simulink model "COSTEP_Auto"  (R2024b)
settings: Solver=FixedStepAuto  StartTime=0.0  StopTime=25  FixedStep=1/3600  RelTol=1e-3
model workspace (MAT data in the model file):
  AD : Simulink.Parameter (value not decoded)
  AG : Simulink.Parameter (value not decoded)
  AH : Simulink.Parameter (value not decoded)
  AV : Simulink.Parameter (value not decoded)
  AVP : Simulink.Parameter (value not decoded)
  BCHL : Simulink.Parameter (value not decoded)
  BCHV : Simulink.Parameter (value not decoded)
  BD : Simulink.Parameter (value not decoded)
  BG : Simulink.Parameter (value not decoded)
  BH : Simulink.Parameter (value not decoded)
  BVP : Simulink.Parameter (value not decoded)
  CD : Simulink.Parameter (value not decoded)
  CG : Simulink.Parameter (value not decoded)
  CH : Simulink.Parameter (value not decoded)
  CVP : Simulink.Parameter (value not decoded)
  ISV : Simulink.Parameter (value not decoded)
  XMW : Simulink.Parameter (value not decoded)
  XNS : Simulink.Parameter (value not decoded)
  XNS2 : Simulink.Parameter (value not decoded)
  XNS3 : Simulink.Parameter (value not decoded)
  XNSE : Simulink.Parameter (value not decoded)
values from neighbouring files (symbols this model uses):
  DD = SimData{4,1}{1,2}    [Auto_run_COSTEP.m]    (also in Run_COSTEP.m)
  G = SimData{2,1}(j,2)    [Auto_run_COSTEP.m]    (also in G.mat = [4243534565 7854912354 3456432354 1731738903 4346024432 5784; Run_COSTEP.m)
  IDV = SimData{3,1}(1:20,j)    [Auto_run_COSTEP.m]    (also in IDV.mat = [0 0 0 0 0 0 0 0 0 0 0 0 ... (812 elements, 28x29)]; Run_COSTEP.m = SimData{3,1}(1:28,j))
symbols that are objects in the model workspace (value not decoded): AD, AG, AH, AV, AVP, BD, BG, BH, BVP, CD, CG, CH, CVP, XMW, XNS, XNS2, XNS3, XNSE
undefined symbols (not defined in the file or in its folder): magnitude, msgbox, SETPT, XMEAS, XMV
libraries: mylib x304, dspindex x31
(part 8 of 13)

== system COSTEP_Auto/Mixing Zone/Stream 6/Subsystem/If Action Subsystem1 ==
  In1 : Inport
  Action Port : ActionPort  ActionPortLabel=else
  Out1 : Outport  VectorParamsAs1DForOutWhenUnconnected=off
  wires:
  In1/1 -> Out1/1

== system COSTEP_Auto/Process Measurements/Feed Streams/D Feed/XMWS(1) Molecular weight of Stream 1 lb//lb-mol ==
  XST(I,1) : Inport
  Product : Product
  Sum of Elements : Sum  Inputs=+
  "XMW(I) Molecular weight of components lb/lb-mol " : Constant  Value=XMW
  XMWS(1) : Outport  VectorParamsAs1DForOutWhenUnconnected=off
  wires:
  Sum of Elements/1 -> XMWS(1)/1
  Product/1 -> Sum of Elements/1
  XST(I,1)/1 -> Product/1
  "XMW(I) Molecular weight of components lb/lb-mol "/1 -> Product/2

== system COSTEP_Auto/Process Measurements/Feed Streams/E Feed/XMWS(2) Molecular weight of Stream 2 lb//lb-mol ==
  XST(I,2) : Inport
  Product : Product
  Sum of Elements : Sum  Inputs=+
  "XMW(I) Molecular weight of components lb/lb-mol " : Constant  Value=XMW
  XMWS(2) : Outport  VectorParamsAs1DForOutWhenUnconnected=off
  wires:
  Sum of Elements/1 -> XMWS(2)/1
  Product/1 -> Sum of Elements/1
  XST(I,2)/1 -> Product/1
  "XMW(I) Molecular weight of components lb/lb-mol "/1 -> Product/2

== system COSTEP_Auto/Process Measurements/Product analysis/Subsystem/Subsystem ==
  XST : Inport
  Constant : Constant  Value=100
  Multiport Selector : dspindex/Multiport Selector  rowsOrCols=Rows  idxCellArray={4,5,6,7,8}  idxErrMode=Clip Index
  XCMP(37) : Product
  XCMP(38) : Product
  XCMP(39) : Product
  XCMP(40) : Product
  XCMP(41) : Product
  "XCMP(37) " : Outport  VectorParamsAs1DForOutWhenUnconnected=off
  "XCMP(38) " : Outport  Port=2  VectorParamsAs1DForOutWhenUnconnected=off
  "XCMP(39) " : Outport  Port=3  VectorParamsAs1DForOutWhenUnconnected=off
  "XCMP(40) " : Outport  Port=4  VectorParamsAs1DForOutWhenUnconnected=off
  "XCMP(41) " : Outport  Port=5  VectorParamsAs1DForOutWhenUnconnected=off
  wires:
  Constant/1 -> XCMP(38)/2, XCMP(40)/2, XCMP(41)/2, XCMP(39)/2, XCMP(37)/2
  Multiport Selector/1 -> XCMP(37)/1
  XCMP(37)/1 -> "XCMP(37) "/1  "XCMP(37)"
  Multiport Selector/5 -> XCMP(41)/1
  XCMP(39)/1 -> "XCMP(39) "/1  "XCMP(39)"
  XST/1 -> Multiport Selector/1
  Multiport Selector/4 -> XCMP(40)/1
  Multiport Selector/2 -> XCMP(38)/1
  Multiport Selector/3 -> XCMP(39)/1
  XCMP(38)/1 -> "XCMP(38) "/1  "XCMP(38)"
  XCMP(41)/1 -> "XCMP(41) "/1  "XCMP(41)"
  XCMP(40)/1 -> "XCMP(40) "/1  "XCMP(40)"

== system COSTEP_Auto/Process Measurements/Purge gas analysis/Subsystem/Subsystem ==
  XST : Inport
  Constant : Constant  Value=100
  Multiport Selector : dspindex/Multiport Selector  rowsOrCols=Rows  idxCellArray={ 1,2,3,4,5,6,7,8}  idxErrMode=Clip Index
  XCMP(29) : Product
  XCMP(30) : Product
  XCMP(31) : Product
  XCMP(32) : Product
  XCMP(33) : Product
  XCMP(34) : Product
  XCMP(35) : Product
  XCMP(36) : Product
  "XCMP(29) " : Outport  VectorParamsAs1DForOutWhenUnconnected=off
  "XCMP(30) " : Outport  Port=2  VectorParamsAs1DForOutWhenUnconnected=off
  "XCMP(31) " : Outport  Port=3  VectorParamsAs1DForOutWhenUnconnected=off
  "XCMP(32) " : Outport  Port=4  VectorParamsAs1DForOutWhenUnconnected=off
  "XCMP(33) " : Outport  Port=5  VectorParamsAs1DForOutWhenUnconnected=off
  "XCMP(34) " : Outport  Port=6  VectorParamsAs1DForOutWhenUnconnected=off
  "XCMP(35) " : Outport  Port=7  VectorParamsAs1DForOutWhenUnconnected=off
  "XCMP(36) " : Outport  Port=8  VectorParamsAs1DForOutWhenUnconnected=off
  wires:
  XCMP(32)/1 -> "XCMP(32) "/1  "XCMP(32)"
  Multiport Selector/6 -> XCMP(34)/1
  Multiport Selector/8 -> XCMP(36)/1
  XCMP(29)/1 -> "XCMP(29) "/1  "XCMP(29)"
  Multiport Selector/5 -> XCMP(33)/1
  Multiport Selector/7 -> XCMP(35)/1
  XCMP(30)/1 -> "XCMP(30) "/1  "XCMP(30)"
  Multiport Selector/1 -> XCMP(29)/1
  Multiport Selector/3 -> XCMP(31)/1
  Constant/1 -> XCMP(32)/2, XCMP(36)/2, XCMP(35)/2, XCMP(34)/2, XCMP(33)/2, XCMP(31)/2, XCMP(30)/2, XCMP(29)/2
  XCMP(33)/1 -> "XCMP(33) "/1  "XCMP(33)"
  Multiport Selector/4 -> XCMP(32)/1
  XST/1 -> Multiport Selector/1
  Multiport Selector/2 -> XCMP(30)/1
  XCMP(31)/1 -> "XCMP(31) "/1  "XCMP(31)"
  XCMP(35)/1 -> "XCMP(35) "/1  "XCMP(35)"
  XCMP(36)/1 -> "XCMP(36) "/1  "XCMP(36)"
  XCMP(34)/1 -> "XCMP(34) "/1  "XCMP(34)"

== system COSTEP_Auto/Process Measurements/Reactor feed analysis/Subsystem/Subsystem ==
  XST : Inport
  Constant : Constant  Value=100
  Multiport Selector : dspindex/Multiport Selector  rowsOrCols=Rows  idxCellArray={ 1,2,3,4,5,6,}  idxErrMode=Clip Index
  XCMP(23) : Product
  XCMP(24) : Product
  XCMP(25) : Product
  XCMP(26) : Product
  XCMP(27) : Product
  XCMP(28) : Product
  XCMP(23)1 : Outport  VectorParamsAs1DForOutWhenUnconnected=off
  XCMP(24)1 : Outport  Port=2  VectorParamsAs1DForOutWhenUnconnected=off
  XCMP(25)1 : Outport  Port=3  VectorParamsAs1DForOutWhenUnconnected=off
  XCMP(26)1 : Outport  Port=4  VectorParamsAs1DForOutWhenUnconnected=off
  XCMP(27)1 : Outport  Port=5  VectorParamsAs1DForOutWhenUnconnected=off
  XCMP(28)1 : Outport  Port=6  VectorParamsAs1DForOutWhenUnconnected=off
  wires:
  Multiport Selector/1 -> XCMP(23)/1  "XST(1;7)"
  Multiport Selector/4 -> XCMP(26)/1  "XST(4;7)"
  Constant/1 -> XCMP(26)/2, XCMP(28)/2, XCMP(27)/2, XCMP(25)/2, XCMP(24)/2, XCMP(23)/2
  Multiport Selector/2 -> XCMP(24)/1  "XST(2;7)"
  XST/1 -> Multiport Selector/1
  Multiport Selector/6 -> XCMP(28)/1  "XST(6:7)"
  Multiport Selector/3 -> XCMP(25)/1  "XST(3;7)"
  XCMP(23)/1 -> XCMP(23)1/1  "XCMP(23)"
  Multiport Selector/5 -> XCMP(27)/1  "XST(5;7)"
  XCMP(25)/1 -> XCMP(25)1/1  "XCMP(25)"
  XCMP(26)/1 -> XCMP(26)1/1  "XCMP(26)"
  XCMP(24)/1 -> XCMP(24)1/1  "XCMP(24)"
  XCMP(27)/1 -> XCMP(27)1/1  "XCMP(27)"
  XCMP(28)/1 -> XCMP(28)1/1  "XCMP(28)"

== system COSTEP_Auto/Random number generator/Disturbances I=1-9/Subsystem1/DIST(2)_0 ==
  BDIST(2) : Constant  Value=0
  Bus Creator : BusCreator  Inputs=6
  CDIST(2) : Constant  Value=0
  DDIST(2) : Constant  Value=0
  SZERO(2) : Constant  Value=0.005
  TENXT(2) : Constant  Value=0.1
  TLAST(2) : Constant  Value=0
  DIST : Outport  VectorParamsAs1DForOutWhenUnconnected=off
  wires:
  Bus Creator/1 -> DIST/1
  TENXT(2)/1 -> Bus Creator/5  "TNEXT"
  SZERO(2)/1 -> Bus Creator/1  "ADIST"
  TLAST(2)/1 -> Bus Creator/6  "TLAST"
  DDIST(2)/1 -> Bus Creator/4  "DDIST"
  BDIST(2)/1 -> Bus Creator/2  "BDIST"
  CDIST(2)/1 -> Bus Creator/3  "CDIST"

== system COSTEP_Auto/Random number generator/Disturbances I=1-9/Subsystem1/Subsystem ==
  Bus Creator : BusCreator  Inputs=5
  HSPAN(2) : Constant  Value=0.7
  HZERO(2) : Constant
  SPSPAN(2) : Constant  Value=0
  SSPAN(2) : Constant  Value=0.003
  SZERO(2) : Constant  Value=0.005
  Out1 : Outport  VectorParamsAs1DForOutWhenUnconnected=off
  wires:
  SSPAN(2)/1 -> Bus Creator/3  "SSPAN"
  HSPAN(2)/1 -> Bus Creator/1  "HSPAN"
  Bus Creator/1 -> Out1/1
  SPSPAN(2)/1 -> Bus Creator/5  "SPSPAN"
  HZERO(2)/1 -> Bus Creator/2  "HZERO"
  SZERO(2)/1 -> Bus Creator/4  "SZERO"

== system COSTEP_Auto/Random number generator/Disturbances I=1-9/Subsystem10/DIST(1)_0 ==
  BDIST(1) : Constant  Value=0
  Bus Creator : BusCreator  Inputs=6
  CDIST(1) : Constant  Value=0
  DDIST(1) : Constant  Value=0
  SZERO(1) : Constant  Value=0.485
  TENXT(1) : Constant  Value=0.1
  TLAST(1) : Constant  Value=0
  DIST : Outport  VectorParamsAs1DForOutWhenUnconnected=off
  wires:
  Bus Creator/1 -> DIST/1
  TENXT(1)/1 -> Bus Creator/5  "TNEXT"
  SZERO(1)/1 -> Bus Creator/1  "ADIST"
  TLAST(1)/1 -> Bus Creator/6  "TLAST"
  DDIST(1)/1 -> Bus Creator/4  "DDIST"
  BDIST(1)/1 -> Bus Creator/2  "BDIST"
  CDIST(1)/1 -> Bus Creator/3  "CDIST"

== system COSTEP_Auto/Random number generator/Disturbances I=1-9/Subsystem10/Subsystem ==
  Bus Creator : BusCreator  Inputs=5
  HSPAN(1) : Constant  Value=0.2
  HZERO(1) : Constant  Value=0.5
  SPSPAN(1) : Constant  Value=0
  SSPAN(1) : Constant  Value=0.03
  SZERO(1) : Constant  Value=0.485
  Out1 : Outport  VectorParamsAs1DForOutWhenUnconnected=off
  wires:
  SSPAN(1)/1 -> Bus Creator/3  "SSPAN"
  HSPAN(1)/1 -> Bus Creator/1  "HSPAN"
  Bus Creator/1 -> Out1/1
  SPSPAN(1)/1 -> Bus Creator/5  "SPSPAN"
  HZERO(1)/1 -> Bus Creator/2  "HZERO"
  SZERO(1)/1 -> Bus Creator/4  "SZERO"

== system COSTEP_Auto/Random number generator/Disturbances I=1-9/Subsystem2/DIST(3)_0 ==
  BDIST(3) : Constant  Value=0
  Bus Creator : BusCreator  Inputs=6
  CDIST(3) : Constant  Value=0
  DDIST(3) : Constant  Value=0
  SZERO(3) : Constant  Value=45
  TENXT(3) : Constant  Value=0.1
  TLAST(3) : Constant  Value=0
  DIST : Outport  VectorParamsAs1DForOutWhenUnconnected=off
  wires:
  Bus Creator/1 -> DIST/1
  TENXT(3)/1 -> Bus Creator/5  "TNEXT"
  SZERO(3)/1 -> Bus Creator/1  "ADIST"
  TLAST(3)/1 -> Bus Creator/6  "TLAST"
  DDIST(3)/1 -> Bus Creator/4  "DDIST"
  BDIST(3)/1 -> Bus Creator/2  "BDIST"
  CDIST(3)/1 -> Bus Creator/3  "CDIST"

== system COSTEP_Auto/Random number generator/Disturbances I=1-9/Subsystem2/Subsystem ==
  Bus Creator : BusCreator  Inputs=5
  HSPAN(3) : Constant  Value=0.25
  HZERO(3) : Constant  Value=0.5
  SPSPAN(3) : Constant  Value=0
  SSPAN(3) : Constant  Value=10
  SZERO(3) : Constant  Value=45
  Out1 : Outport  VectorParamsAs1DForOutWhenUnconnected=off
  wires:
  SSPAN(3)/1 -> Bus Creator/3  "SSPAN"
  HSPAN(3)/1 -> Bus Creator/1  "HSPAN"
  Bus Creator/1 -> Out1/1
  SPSPAN(3)/1 -> Bus Creator/5  "SPSPAN"
  HZERO(3)/1 -> Bus Creator/2  "HZERO"
  SZERO(3)/1 -> Bus Creator/4  "SZERO"

== system COSTEP_Auto/Random number generator/Disturbances I=1-9/Subsystem3/DIST(4)_0 ==
  BDIST(4) : Constant  Value=0
  Bus Creator : BusCreator  Inputs=6
  CDIST(4) : Constant  Value=0
  DDIST(4) : Constant  Value=0
  SZERO(4) : Constant  Value=45
  TENXT(4) : Constant  Value=0.1
  TLAST(4) : Constant  Value=0
  DIST : Outport  VectorParamsAs1DForOutWhenUnconnected=off
  wires:
  Bus Creator/1 -> DIST/1
  TENXT(4)/1 -> Bus Creator/5  "TNEXT"
  SZERO(4)/1 -> Bus Creator/1  "ADIST"
  TLAST(4)/1 -> Bus Creator/6  "TLAST"
  DDIST(4)/1 -> Bus Creator/4  "DDIST"
  BDIST(4)/1 -> Bus Creator/2  "BDIST"
  CDIST(4)/1 -> Bus Creator/3  "CDIST"

== system COSTEP_Auto/Random number generator/Disturbances I=1-9/Subsystem3/Subsystem ==
  Bus Creator : BusCreator  Inputs=5
  HSPAN(4) : Constant  Value=0.7
  HZERO(4) : Constant
  SPSPAN(4) : Constant  Value=0
  SSPAN(4) : Constant  Value=10
  SZERO(4) : Constant  Value=45
  Out1 : Outport  VectorParamsAs1DForOutWhenUnconnected=off
  wires:
  SSPAN(4)/1 -> Bus Creator/3  "SSPAN"
  HSPAN(4)/1 -> Bus Creator/1  "HSPAN"
  Bus Creator/1 -> Out1/1
  SPSPAN(4)/1 -> Bus Creator/5  "SPSPAN"
  HZERO(4)/1 -> Bus Creator/2  "HZERO"
  SZERO(4)/1 -> Bus Creator/4  "SZERO"

== system COSTEP_Auto/Random number generator/Disturbances I=1-9/Subsystem4/DIST(5)_0 ==
  BDIST(5) : Constant  Value=0
  Bus Creator : BusCreator  Inputs=6
  CDIST(5) : Constant  Value=0
  DDIST(5) : Constant  Value=0
  SZERO(5) : Constant  Value=35
  TENXT(5) : Constant  Value=0.1
  TLAST(5) : Constant  Value=0
  DIST : Outport  VectorParamsAs1DForOutWhenUnconnected=off
  wires:
  Bus Creator/1 -> DIST/1
  TENXT(5)/1 -> Bus Creator/5  "TNEXT"
  SZERO(5)/1 -> Bus Creator/1  "ADIST"
  TLAST(5)/1 -> Bus Creator/6  "TLAST"
  DDIST(5)/1 -> Bus Creator/4  "DDIST"
  BDIST(5)/1 -> Bus Creator/2  "BDIST"
  CDIST(5)/1 -> Bus Creator/3  "CDIST"

== system COSTEP_Auto/Random number generator/Disturbances I=1-9/Subsystem4/Subsystem ==
  Bus Creator : BusCreator  Inputs=5
  HSPAN(5) : Constant  Value=0.15
  HZERO(5) : Constant  Value=0.25
  SPSPAN(5) : Constant  Value=0
  SSPAN(5) : Constant  Value=10
  SZERO(5) : Constant  Value=35
  Out1 : Outport  VectorParamsAs1DForOutWhenUnconnected=off
  wires:
  SSPAN(5)/1 -> Bus Creator/3  "SSPAN"
  HSPAN(5)/1 -> Bus Creator/1  "HSPAN"
  Bus Creator/1 -> Out1/1
  SPSPAN(5)/1 -> Bus Creator/5  "SPSPAN"
  HZERO(5)/1 -> Bus Creator/2  "HZERO"
  SZERO(5)/1 -> Bus Creator/4  "SZERO"

== system COSTEP_Auto/Random number generator/Disturbances I=1-9/Subsystem5/DIST(6)_0 ==
  BDIST(6) : Constant  Value=0
  Bus Creator : BusCreator  Inputs=6
  CDIST(6) : Constant  Value=0
  DDIST(6) : Constant  Value=0
  SZERO(6) : Constant  Value=40
  TENXT(6) : Constant  Value=0.1
  TLAST(6) : Constant  Value=0
  DIST : Outport  VectorParamsAs1DForOutWhenUnconnected=off
  wires:
  Bus Creator/1 -> DIST/1
  TENXT(6)/1 -> Bus Creator/5  "TNEXT"
  SZERO(6)/1 -> Bus Creator/1  "ADIST"
  TLAST(6)/1 -> Bus Creator/6  "TLAST"
  DDIST(6)/1 -> Bus Creator/4  "DDIST"
  BDIST(6)/1 -> Bus Creator/2  "BDIST"
  CDIST(6)/1 -> Bus Creator/3  "CDIST"

== system COSTEP_Auto/Random number generator/Disturbances I=1-9/Subsystem5/Subsystem ==
  Bus Creator : BusCreator  Inputs=5
  HSPAN(6) : Constant  Value=0.15
  HZERO(6) : Constant  Value=0.25
  SPSPAN(6) : Constant  Value=0
  SSPAN(6) : Constant  Value=10
  SZERO(6) : Constant  Value=40
  Out1 : Outport  VectorParamsAs1DForOutWhenUnconnected=off
  wires:
  SSPAN(6)/1 -> Bus Creator/3  "SSPAN"
  HSPAN(6)/1 -> Bus Creator/1  "HSPAN"
  Bus Creator/1 -> Out1/1
  SPSPAN(6)/1 -> Bus Creator/5  "SPSPAN"
  HZERO(6)/1 -> Bus Creator/2  "HZERO"
  SZERO(6)/1 -> Bus Creator/4  "SZERO"

== system COSTEP_Auto/Random number generator/Disturbances I=1-9/Subsystem6/DIST(7)_0 ==
  BDIST(7) : Constant  Value=0
  Bus Creator : BusCreator  Inputs=6
  CDIST(7) : Constant  Value=0
  DDIST(7) : Constant  Value=0
  SZERO(7) : Constant
  TENXT(7) : Constant  Value=0.1
  TLAST(7) : Constant  Value=0
  DIST : Outport  VectorParamsAs1DForOutWhenUnconnected=off
  wires:
  Bus Creator/1 -> DIST/1
  TENXT(7)/1 -> Bus Creator/5  "TNEXT"
  SZERO(7)/1 -> Bus Creator/1  "ADIST"
  TLAST(7)/1 -> Bus Creator/6  "TLAST"
  DDIST(7)/1 -> Bus Creator/4  "DDIST"
  BDIST(7)/1 -> Bus Creator/2  "BDIST"
  CDIST(7)/1 -> Bus Creator/3  "CDIST"

== system COSTEP_Auto/Random number generator/Disturbances I=1-9/Subsystem6/Subsystem ==
  Bus Creator : BusCreator  Inputs=5
  HSPAN(7) : Constant
  HZERO(7) : Constant  Value=2
  SPSPAN(7) : Constant  Value=0
  SSPAN(7) : Constant  Value=0.25
  SZERO(7) : Constant
  Out1 : Outport  VectorParamsAs1DForOutWhenUnconnected=off
  wires:
  SSPAN(7)/1 -> Bus Creator/3  "SSPAN"
  HSPAN(7)/1 -> Bus Creator/1  "HSPAN"
  Bus Creator/1 -> Out1/1
  SPSPAN(7)/1 -> Bus Creator/5  "SPSPAN"
  HZERO(7)/1 -> Bus Creator/2  "HZERO"
  SZERO(7)/1 -> Bus Creator/4  "SZERO"

== system COSTEP_Auto/Random number generator/Disturbances I=1-9/Subsystem7/DIST(8)_0 ==
  BDIST(8) : Constant  Value=0
  Bus Creator : BusCreator  Inputs=6
  CDIST(8) : Constant  Value=0
  DDIST(8) : Constant  Value=0
  SZERO(8) : Constant
  TENXT(8) : Constant  Value=0.1
  TLAST(8) : Constant  Value=0
  DIST : Outport  VectorParamsAs1DForOutWhenUnconnected=off
  wires:
  Bus Creator/1 -> DIST/1
  TENXT(8)/1 -> Bus Creator/5  "TNEXT"
  SZERO(8)/1 -> Bus Creator/1  "ADIST"
  TLAST(8)/1 -> Bus Creator/6  "TLAST"
  DDIST(8)/1 -> Bus Creator/4  "DDIST"
  BDIST(8)/1 -> Bus Creator/2  "BDIST"
  CDIST(8)/1 -> Bus Creator/3  "CDIST"

== system COSTEP_Auto/Random number generator/Disturbances I=1-9/Subsystem7/Subsystem ==
  Bus Creator : BusCreator  Inputs=5
  HSPAN(8) : Constant
  HZERO(8) : Constant  Value=2
  SPSPAN(8) : Constant  Value=0
  SSPAN(8) : Constant  Value=0.25
  SZERO(8) : Constant
  Out1 : Outport  VectorParamsAs1DForOutWhenUnconnected=off
  wires:
  SSPAN(8)/1 -> Bus Creator/3  "SSPAN"
  HSPAN(8)/1 -> Bus Creator/1  "HSPAN"
  Bus Creator/1 -> Out1/1
  SPSPAN(8)/1 -> Bus Creator/5  "SPSPAN"
  HZERO(8)/1 -> Bus Creator/2  "HZERO"
  SZERO(8)/1 -> Bus Creator/4  "SZERO"

== system COSTEP_Auto/Random number generator/Disturbances I=1-9/Subsystem8/DIST(9)_0 ==
  BDIST(9) : Constant  Value=0
  Bus Creator : BusCreator  Inputs=6
  CDIST(9) : Constant  Value=0
  DDIST(9) : Constant  Value=0
  SZERO(9) : Constant  Value=0
  TENXT(9) : Constant  Value=0.1
  TLAST(9) : Constant  Value=0
  DIST : Outport  VectorParamsAs1DForOutWhenUnconnected=off
  wires:
  Bus Creator/1 -> DIST/1
  TENXT(9)/1 -> Bus Creator/5  "TNEXT"
  SZERO(9)/1 -> Bus Creator/1  "ADIST"
  TLAST(9)/1 -> Bus Creator/6  "TLAST"
  DDIST(9)/1 -> Bus Creator/4  "DDIST"
  BDIST(9)/1 -> Bus Creator/2  "BDIST"
  CDIST(9)/1 -> Bus Creator/3  "CDIST"

== system COSTEP_Auto/Random number generator/Disturbances I=1-9/Subsystem8/Subsystem ==
  Bus Creator : BusCreator  Inputs=5
  HSPAN(9) : Constant  Value=0.4
  HZERO(9) : Constant  Value=0.5
  SPSPAN(9) : Constant  Value=0
  SSPAN(9) : Constant  Value=0.25
  SZERO(9) : Constant  Value=0
  Out1 : Outport  VectorParamsAs1DForOutWhenUnconnected=off
  wires:
  SSPAN(9)/1 -> Bus Creator/3  "SSPAN"
  HSPAN(9)/1 -> Bus Creator/1  "HSPAN"
  Bus Creator/1 -> Out1/1
  SPSPAN(9)/1 -> Bus Creator/5  "SPSPAN"
  HZERO(9)/1 -> Bus Creator/2  "HZERO"
  SZERO(9)/1 -> Bus Creator/4  "SZERO"

== system COSTEP_Auto/Random number generator/Disturbances I=10-12/Subsystem1/DIST(11)_0 ==
  BDIST(11) : Constant  Value=0
  Bus Creator : BusCreator  Inputs=6
  CDIST(11) : Constant  Value=0
  DDIST(11) : Constant  Value=0
  SZERO(11) : Constant  Value=0
  TENXT(11) : Constant  Value=0.1
  TLAST(11) : Constant  Value=0
  DIST_0 : Outport  VectorParamsAs1DForOutWhenUnconnected=off
  wires:
  Bus Creator/1 -> DIST_0/1
  TENXT(11)/1 -> Bus Creator/5  "TNEXT"
  SZERO(11)/1 -> Bus Creator/1  "ADIST"
  TLAST(11)/1 -> Bus Creator/6  "TLAST"
  DDIST(11)/1 -> Bus Creator/4  "DDIST"
  BDIST(11)/1 -> Bus Creator/2  "BDIST"
  CDIST(11)/1 -> Bus Creator/3  "CDIST"

== system COSTEP_Auto/Random number generator/Disturbances I=10-12/Subsystem1/Subsystem2 ==
  Bus Creator : BusCreator  Inputs=5
  HSPAN(11) : Constant  Value=2
  HZERO(11) : Constant  Value=3
  SPSPAN(11) : Constant  Value=0
  SSPAN(11) : Constant  Value=0
  SZERO(11) : Constant  Value=0
  Out1 : Outport  VectorParamsAs1DForOutWhenUnconnected=off
  wires:
  SSPAN(11)/1 -> Bus Creator/3  "SSPAN"
  HSPAN(11)/1 -> Bus Creator/1  "HSPAN"
  Bus Creator/1 -> Out1/1
  SPSPAN(11)/1 -> Bus Creator/5  "SPSPAN"
  HZERO(11)/1 -> Bus Creator/2  "HZERO"
  SZERO(11)/1 -> Bus Creator/4  "SZERO"

== system COSTEP_Auto/Random number generator/Disturbances I=10-12/Subsystem10/DIST(10)_0 ==
  BDIST(10) : Constant  Value=0
  Bus Creator1 : BusCreator  Inputs=6
  CDIST(10) : Constant  Value=0
  DDIST(10) : Constant  Value=0
  SZERO(10) : Constant  Value=0
  TENXT(10) : Constant  Value=0.1
  TLAST(10) : Constant  Value=0
  DIST_0 : Outport  VectorParamsAs1DForOutWhenUnconnected=off
  wires:
  TENXT(10)/1 -> Bus Creator1/5  "TNEXT"
  DDIST(10)/1 -> Bus Creator1/4  "DDIST"
  TLAST(10)/1 -> Bus Creator1/6  "TLAST"
  SZERO(10)/1 -> Bus Creator1/1  "ADIST"
  CDIST(10)/1 -> Bus Creator1/3  "CDIST"
  BDIST(10)/1 -> Bus Creator1/2  "BDIST"
  Bus Creator1/1 -> DIST_0/1

== system COSTEP_Auto/Random number generator/Disturbances I=10-12/Subsystem10/Subsystem2 ==
  Bus Creator : BusCreator  Inputs=5
  HSPAN(10) : Constant  Value=1.5
  HZERO(10) : Constant  Value=2
  SPSPAN(10) : Constant  Value=0
  SSPAN(10) : Constant  Value=0
  SZERO(10) : Constant  Value=0
  Out1 : Outport  VectorParamsAs1DForOutWhenUnconnected=off
  wires:
  SSPAN(10)/1 -> Bus Creator/3  "SSPAN"
  HSPAN(10)/1 -> Bus Creator/1  "HSPAN"
  Bus Creator/1 -> Out1/1
  SPSPAN(10)/1 -> Bus Creator/5  "SPSPAN"
  HZERO(10)/1 -> Bus Creator/2  "HZERO"
  SZERO(10)/1 -> Bus Creator/4  "SZERO"

== system COSTEP_Auto/Random number generator/Disturbances I=10-12/Subsystem2/DIST(12)_0 ==
  BDIST(12) : Constant  Value=0
  Bus Creator : BusCreator  Inputs=6
  CDIST(12) : Constant  Value=0
  DDIST(12) : Constant  Value=0
  SZERO(12) : Constant  Value=0
  TENXT(12) : Constant  Value=0.1
  TLAST(12) : Constant  Value=0
  DIST_0 : Outport  VectorParamsAs1DForOutWhenUnconnected=off
  wires:
  Bus Creator/1 -> DIST_0/1
  TENXT(12)/1 -> Bus Creator/5  "TNEXT"
  SZERO(12)/1 -> Bus Creator/1  "ADIST"
  TLAST(12)/1 -> Bus Creator/6  "TLAST"
  DDIST(12)/1 -> Bus Creator/4  "DDIST"
  BDIST(12)/1 -> Bus Creator/2  "BDIST"
  CDIST(12)/1 -> Bus Creator/3  "CDIST"

== system COSTEP_Auto/Random number generator/Disturbances I=10-12/Subsystem2/Subsystem2 ==
  Bus Creator : BusCreator  Inputs=5
  HSPAN(12) : Constant  Value=1.5
  HZERO(12) : Constant  Value=2
  SPSPAN(12) : Constant  Value=0
  SSPAN(12) : Constant  Value=0
  SZERO(12) : Constant  Value=0
  Out1 : Outport  VectorParamsAs1DForOutWhenUnconnected=off
  wires:
  SSPAN(12)/1 -> Bus Creator/3  "SSPAN"
  HSPAN(12)/1 -> Bus Creator/1  "HSPAN"
  Bus Creator/1 -> Out1/1
  SPSPAN(12)/1 -> Bus Creator/5  "SPSPAN"
  HZERO(12)/1 -> Bus Creator/2  "HZERO"
  SZERO(12)/1 -> Bus Creator/4  "SZERO"

== system COSTEP_Auto/Random number generator/Stream Measurements SMEAS Gas analysis/Gas Analysis Delay/Subsystem ==
  In1 : Inport
  In2 : Inport  Port=2
  If : If  NumInputs=2  IfExpression=u1 == u2
  If Action Subsystem : Subsystem  TreatAsAtomicUnit=on
  If Action Subsystem1 : Subsystem  TreatAsAtomicUnit=on
  Rounding Function : Rounding  Operator=round
  Out1 : Outport  VectorParamsAs1DForOutWhenUnconnected=off
  Out2 : Outport  Port=2  VectorParamsAs1DForOutWhenUnconnected=off
  wires:
  Rounding Function/1 -> If/1, If Action Subsystem1/1(In1)
  In2/1 -> If/2
  If Action Subsystem/1(Out1) -> Out1/1
  If Action Subsystem1/1(Out1) -> Out2/1
  In1/1 -> Rounding Function/1
  If/1 -> If Action Subsystem/Action
  If/2 -> If Action Subsystem1/Action

== system COSTEP_Auto/Random number generator/Stream Measurements SMEAS Gas analysis/If Action Subsystem3/Subsystem ==
  G : Inport
  Bus Creator2 : BusCreator  Inputs=9
  Stream 1 : Subsystem
  Stream 13 : Subsystem
  Stream 2 : Subsystem
  Stream 3 : Subsystem
  Stream 4 : Subsystem
  Stream 5 : Subsystem
  Stream 6 : Subsystem
  Stream 8 : Subsystem
  Stream 9 : Subsystem
  XMNSE2 : Outport  VectorParamsAs1DForOutWhenUnconnected=off
  G_NEW : Outport  Port=2  VectorParamsAs1DForOutWhenUnconnected=off
  wires:
  Bus Creator2/1 -> XMNSE2/1
  G/1 -> Stream 1/1(G)
  Stream 1/1(Stream 1) -> Bus Creator2/1
  Stream 1/2(G_NEW) -> Stream 2/1(G)
  Stream 2/1(Stream 2) -> Bus Creator2/2
  Stream 2/2(G_NEW) -> Stream 3/1(G)
  Stream 3/1(Stream 3) -> Bus Creator2/3
  Stream 3/2(G_NEW) -> Stream 4/1(G)
  Stream 4/1(Stream 4) -> Bus Creator2/4
  Stream 4/2(G_NEW) -> Stream 5/1(G)
  Stream 5/1(Stream 5) -> Bus Creator2/5
  Stream 5/2(G_NEW) -> Stream 6/1(G)
  Stream 6/1(Stream 6) -> Bus Creator2/6
  Stream 6/2(G_NEW) -> Stream 8/1(G)
  Stream 8/1(Stream 8) -> Bus Creator2/7
  Stream 8/2(G_NEW) -> Stream 9/1(G)
  Stream 9/1(Stream 9) -> Bus Creator2/8
  Stream 9/2(G_NEW) -> Stream 13/1(G)
  Stream 13/2(G_NEW) -> G_NEW/1
  Stream 13/1(Stream 13) -> Bus Creator2/9

== system COSTEP_Auto/Random number generator/Stream Measurements SMEAS Gas analysis/Subsystem/If Action Subsystem ==
  In1 : Inport
  Action Port : ActionPort  ActionPortLabel=if(u1 == 0)
  Out1 : Outport  VectorParamsAs1DForOutWhenUnconnected=off
  wires:
  In1/1 -> Out1/1

== system COSTEP_Auto/Random number generator/Stream Measurements SMEAS Gas analysis/Subsystem/If Action Subsystem1 ==
  In1 : Inport
  Action Port : ActionPort  ActionPortLabel=else
  Out1 : Outport  VectorParamsAs1DForOutWhenUnconnected=off
  wires:
  In1/1 -> Out1/1

== system COSTEP_Auto/Random number generator/Stream Measurements SMEAS Product analysis/Gas Analysis Delay/Subsystem ==
  In1 : Inport
  In2 : Inport  Port=2
  If : If  NumInputs=2  IfExpression=u1 == u2
  If Action Subsystem : Subsystem  TreatAsAtomicUnit=on
  If Action Subsystem1 : Subsystem  TreatAsAtomicUnit=on
  Rounding Function : Rounding  Operator=round
  Out1 : Outport  VectorParamsAs1DForOutWhenUnconnected=off
  Out2 : Outport  Port=2  VectorParamsAs1DForOutWhenUnconnected=off
  wires:
  Rounding Function/1 -> If/1, If Action Subsystem1/1(In1)
  In2/1 -> If/2
  If Action Subsystem/1(Out1) -> Out1/1
  If Action Subsystem1/1(Out1) -> Out2/1
  In1/1 -> Rounding Function/1
  If/1 -> If Action Subsystem/Action
  If/2 -> If Action Subsystem1/Action

== system COSTEP_Auto/Random number generator/Stream Measurements SMEAS Product analysis/If Action Subsystem3/Subsystem ==
  G : Inport
  Bus Creator : BusCreator  Inputs=2
  Subsystem1 : Subsystem
  Subsystem2 : Subsystem
  XMNSE3 : Outport  VectorParamsAs1DForOutWhenUnconnected=off
  G_NEW : Outport  Port=2  VectorParamsAs1DForOutWhenUnconnected=off
  wires:
  G/1 -> Subsystem1/1(G)
  Subsystem1/1(Stream 11) -> Bus Creator/1
  Bus Creator/1 -> XMNSE3/1
  Subsystem1/2(G_NEW) -> Subsystem2/1(G)
  Subsystem2/1(Stream 13) -> Bus Creator/2
  Subsystem2/2(G_NEW) -> G_NEW/1

== system COSTEP_Auto/Random number generator/Stream Measurements SMEAS Product analysis/Subsystem/If Action Subsystem ==
  In1 : Inport
  Action Port : ActionPort  ActionPortLabel=if(u1 == 0)
  Out1 : Outport  VectorParamsAs1DForOutWhenUnconnected=off
  wires:
  In1/1 -> Out1/1

== system COSTEP_Auto/Random number generator/Stream Measurements SMEAS Product analysis/Subsystem/If Action Subsystem1 ==
  In1 : Inport
  Action Port : ActionPort  ActionPortLabel=else
  Out1 : Outport  VectorParamsAs1DForOutWhenUnconnected=off
  wires:
  In1/1 -> Out1/1

== system COSTEP_Auto/Reactor/Reaction Rates/Component reaction rate lb-mol//h/Subsystem ==
  RR : Inport
  " " : Sum  Inputs=---
  Bus Selector : BusSelector  OutputSignals=RR(1),RR(2),RR(3)
  CRXR(1) : Outport  VectorParamsAs1DForOutWhenUnconnected=off
  wires:
  " "/1 -> CRXR(1)/1  "CRXR(1)"
  Bus Selector/2 -> " "/2  "<RR(2)>"
  Bus Selector/3 -> " "/3  "<RR(3)>"
  RR/1 -> Bus Selector/1
  Bus Selector/1 -> " "/1  "<RR(1)>"

== system COSTEP_Auto/Reactor/Reaction Rates/Component reaction rate lb-mol//h/Subsystem1 ==
  RR : Inport
  " " : Sum  Inputs=--
  Bus Selector : BusSelector  OutputSignals=RR(1),RR(2)
  CRXR(3) : Outport  VectorParamsAs1DForOutWhenUnconnected=off
  wires:
  " "/1 -> CRXR(3)/1  "CRXR(3)"
  RR/1 -> Bus Selector/1
  Bus Selector/1 -> " "/1  "<RR(1)>"
  Bus Selector/2 -> " "/2  "<RR(2)>"

== system COSTEP_Auto/Reactor/Reaction Rates/Component reaction rate lb-mol//h/Subsystem2 ==
  RR : Inport
  " " : Sum  Inputs=--
  Bus Selector : BusSelector  OutputSignals=RR(1),RR(4)
  Gain : Gain  Gain=1.5
  CRXR(4) : Outport  VectorParamsAs1DForOutWhenUnconnected=off
  wires:
  Gain/1 -> " "/2
  Bus Selector/1 -> " "/1  "<RR(1)>"
  " "/1 -> CRXR(4)/1  "CRXR(4)"
  RR/1 -> Bus Selector/1
  Bus Selector/2 -> Gain/1  "<RR(4)>"

== system COSTEP_Auto/Reactor/Reaction Rates/Component reaction rate lb-mol//h/Subsystem3 ==
  RR : Inport
  " " : Sum  Inputs=--
  Bus Selector : BusSelector  OutputSignals=RR(2),RR(3)
  CRXR(5) : Outport  VectorParamsAs1DForOutWhenUnconnected=off
  wires:
  " "/1 -> CRXR(5)/1  "CRXR(5)"
  RR/1 -> Bus Selector/1
  Bus Selector/1 -> " "/1  "<RR(2)>"
  Bus Selector/2 -> " "/2  "<RR(3)>"

== system COSTEP_Auto/Reactor/Reaction Rates/Component reaction rate lb-mol//h/Subsystem4 ==
  RR : Inport
  " " : Sum
  Bus Selector : BusSelector  OutputSignals=RR(3),RR(4)
  CRXR(6) : Outport  VectorParamsAs1DForOutWhenUnconnected=off
  wires:
  " "/1 -> CRXR(6)/1  "CRXR(6)"
  RR/1 -> Bus Selector/1
  Bus Selector/2 -> " "/2  "<RR(4)>"
  Bus Selector/1 -> " "/1  "<RR(3)>"

== system COSTEP_Auto/Reactor/Reaction Rates/Component reaction rate lb-mol//h/Subsystem5 ==
  RR : Inport
  Bus Selector : BusSelector  OutputSignals=RR(1)
  Gain : Gain
  CRXR(7) : Outport  VectorParamsAs1DForOutWhenUnconnected=off
  wires:
  Bus Selector/1 -> Gain/1  "<RR(1)>"
  RR/1 -> Bus Selector/1
  Gain/1 -> CRXR(7)/1  "CRXR(7)"

== system COSTEP_Auto/Reactor/Reaction Rates/Component reaction rate lb-mol//h/Subsystem6 ==
  RR : Inport
  " " : Gain
  Bus Selector : BusSelector  OutputSignals=RR(2)
  CRXR(8) : Outport  VectorParamsAs1DForOutWhenUnconnected=off
  wires:
  " "/1 -> CRXR(8)/1  "CRXR(8)"
  RR/1 -> Bus Selector/1
  Bus Selector/1 -> " "/1  "<RR(2)>"

== system COSTEP_Auto/Reactor/Reaction Rates/Reaction rates lb-mol//h/ Reaction rate of reaction 4 lb-mol//ft3·h     ==
  PPR : Inport
  TKR : Inport  Port=2
  Activation energy cal/mol : Constant  Value=60000
  Bus Selector : BusSelector  OutputSignals=PPR(1),PPR(4)
  Divide : Product  Inputs=*//
  Divide1 : Product  Inputs=3
  Gain : Gain  Gain=0.767488334
  Math Function2 : Math  SignedPower=on
  Preexponential factor lb-mol/ft3·h·mmHg : Constant  Value=53.4060443
  Subtract : Sum  Inputs=+-
  Universal gas constant cal/mol·K : Constant  Value=1.987
  RR(4) : Outport  VectorParamsAs1DForOutWhenUnconnected=off
  wires:
  Divide/1 -> Subtract/2
  Universal gas constant cal/mol·K/1 -> Divide/2
  Preexponential factor lb-mol/ft3·h·mmHg/1 -> Subtract/1
  Activation energy cal/mol/1 -> Divide/1
  TKR/1 -> Divide/3
  Subtract/1 -> Math Function2/1
  Divide1/1 -> RR(4)/1
  Bus Selector/2 -> Divide1/3  "<PPR(4)>"
  Gain/1 -> Divide1/1
  Math Function2/1 -> Gain/1
  PPR/1 -> Bus Selector/1
  Bus Selector/1 -> Divide1/2  "<PPR(1)>"

== system COSTEP_Auto/Reactor/Reaction Rates/Reaction rates lb-mol//h/Reaction rate of reaction 1 lb-mol//ft3·h ==
  PPR : Inport
  TKR : Inport  Port=2
  " " : Constant  Value=0
  Abs : Abs  SaturateOnIntegerOverflow=off
  Bus Selector : BusSelector  OutputSignals=PPR(1),PPR(3)
  If : If  NumInputs=2  IfExpression=u1>0 & u2>0
  If Action Subsystem : Subsystem  TreatAsAtomicUnit=on
  If Action Subsystem2 : Subsystem  TreatAsAtomicUnit=on
  Merge1 : Merge
  "RR(1) Reaction rate of 1st reaction lb-mol/ft3·h " : Subsystem
  RR(1) : Outport  VectorParamsAs1DForOutWhenUnconnected=off
  wires:
  "RR(1) Reaction rate of 1st reaction lb-mol/ft3·h "/1(RR(1)) -> If Action Subsystem/1(In1)
  If/1 -> If Action Subsystem/Action
  " "/1 -> If Action Subsystem2/1(In1)
  If/2 -> If Action Subsystem2/Action
  Merge1/1 -> Abs/1
  If Action Subsystem/1(Out1) -> Merge1/1
  If Action Subsystem2/1(Out1) -> Merge1/2
  TKR/1 -> "RR(1) Reaction rate of 1st reaction lb-mol/ft3·h "/2(TKR)
  Abs/1 -> RR(1)/1
  PPR/1 -> "RR(1) Reaction rate of 1st reaction lb-mol/ft3·h "/1(PPR), Bus Selector/1
  Bus Selector/1 -> If/1  "<PPR(1)>"
  Bus Selector/2 -> If/2  "<PPR(3)>"

== system COSTEP_Auto/Reactor/Reaction Rates/Reaction rates lb-mol//h/Reaction rate of reaction 2 lb-mol//ft3·h ==
  PPR : Inport
  TKR : Inport  Port=2
  " " : Constant  Value=0
  Abs : Abs  SaturateOnIntegerOverflow=off
  Bus Selector : BusSelector  OutputSignals=PPR(1),PPR(3)
  If : If  NumInputs=2  IfExpression=u1>0 & u2>0
  If Action Subsystem : Subsystem  TreatAsAtomicUnit=on
  If Action Subsystem2 : Subsystem  TreatAsAtomicUnit=on
  Merge1 : Merge
  "RR(2) Reaction rate of 2nd reaction lb-mol/ft3·h " : Subsystem
  RR(2) : Outport  VectorParamsAs1DForOutWhenUnconnected=off
  wires:
  If/1 -> If Action Subsystem/Action
  If/2 -> If Action Subsystem2/Action
  "RR(2) Reaction rate of 2nd reaction lb-mol/ft3·h "/1(RR(2)) -> If Action Subsystem/1(In1)
  " "/1 -> If Action Subsystem2/1(In1)
  If Action Subsystem2/1(Out1) -> Merge1/2
  TKR/1 -> "RR(2) Reaction rate of 2nd reaction lb-mol/ft3·h "/2(TKR)
  If Action Subsystem/1(Out1) -> Merge1/1
  Merge1/1 -> Abs/1
  Abs/1 -> RR(2)/1
  PPR/1 -> "RR(2) Reaction rate of 2nd reaction lb-mol/ft3·h "/1(PPR), Bus Selector/1
  Bus Selector/1 -> If/1  "<PPR(1)>"
  Bus Selector/2 -> If/2  "<PPR(3)>"

== system COSTEP_Auto/Reactor/Reaction Rates/Reaction rates lb-mol//h/Reaction rate of reaction 3 lb-mol//ft3·h   ==
  PPR : Inport
  TKR : Inport  Port=2
  Activation energy cal/mol : Constant  Value=60000
  Bus Selector : BusSelector  OutputSignals=PPR(1),PPR(5)
  Divide : Product  Inputs=*//
  Divide1 : Product  Inputs=3
  Math Function2 : Math  SignedPower=on
  Preexponential factor lb-mol/ft3·h·mmHg : Constant  Value=53.4060443
  Subtract : Sum  Inputs=+-
  Universal gas constant cal/mol·K : Constant  Value=1.987
  RR(3) : Outport  VectorParamsAs1DForOutWhenUnconnected=off
  wires:
  Divide/1 -> Subtract/2
  Universal gas constant cal/mol·K/1 -> Divide/2
  Preexponential factor lb-mol/ft3·h·mmHg/1 -> Subtract/1
  Activation energy cal/mol/1 -> Divide/1
  TKR/1 -> Divide/3
  Subtract/1 -> Math Function2/1
  Bus Selector/2 -> Divide1/3  "<PPR(5)>"
  Divide1/1 -> RR(3)/1
  Math Function2/1 -> Divide1/1
  PPR/1 -> Bus Selector/1
  Bus Selector/1 -> Divide1/2  "<PPR(1)>"

== system COSTEP_Auto/Reactor/Reactor Heat exchanger/Position of Valve 12 %/Control valve ==
  XMV(12) : Inport
  Saturation : Saturate  UpperLimit=100  LowerLimit=0
  VCV(12) : Outport  PortDimensions=1  VectorParamsAs1DForOutWhenUnconnected=off
  wires:
  Saturation/1 -> VCV(12)/1
  XMV(12)/1 -> Saturation/1

== system COSTEP_Auto/Reactor/Reactor Heat exchanger/Reactor Heat exchanger/AGSP Agitation speed ==
  VPOS(12) : Inport
  " " : Product  Inputs=*/
  Add : Sum
  Constant1 : Constant  Value=150
  Constant2 : Constant  Value=100
  AGSP : Outport  VectorParamsAs1DForOutWhenUnconnected=off
  wires:
  Constant2/1 -> " "/2
  " "/1 -> AGSP/1
  VPOS(12)/1 -> Add/1
  Constant1/1 -> Add/2
  Add/1 -> " "/1

== system COSTEP_Auto/Reactor/Reactor Heat exchanger/Reactor Heat exchanger/Cooling water outlet temperature ==
  FWR : Inport
  QUR : Inport  Port=2  PortDimensions=1
  Constant1 : Constant  Value=1e6
  Constant2 : Constant  Value=1.8
  Constant6 : Constant  Value=500.53
  Divide : Product  Inputs=*/
  Divide1 : Product
  Divide2 : Product  Inputs=*/
  HWR : Constant  Value=7060
  Integration : mylib/Integration  SystemSampleTime=-1  VariantActivationTime=update diagram  AllowFlexibleInterface=on  Latency=0  AutoFrameSizeCalculation=off
  Product : Product  Inputs=3
  Subtract : Sum  Inputs=+-
  "TCWR Inlet temperature of cooling water °C " : Subsystem
  TCWR-TWR : Sum  Inputs=+-
  YY(37) : Constant  Value=94.59927549
  "YY(37) " : Outport  VectorParamsAs1DForOutWhenUnconnected=off
  tag scope: TCWR=global, TWR=global
  wires:
  Divide2/1 -> Integration/1
  YY(37)/1 -> Integration/2
  "TCWR Inlet temperature of cooling water °C "/1(TCWR) -> [TCWR], TCWR-TWR/1
  Integration/1 -> TCWR-TWR/2, "YY(37) "/1, [TWR]
  FWR/1 -> Product/1
  Constant6/1 -> Product/2
  TCWR-TWR/1 -> Product/3
  QUR/1 -> Divide1/1
  Constant1/1 -> Divide1/2
  Divide1/1 -> Divide/1
  Constant2/1 -> Divide/2
  Product/1 -> Subtract/1
  Divide/1 -> Subtract/2
  Subtract/1 -> Divide2/1
  HWR/1 -> Divide2/2

== system COSTEP_Auto/Reactor/Reactor Heat exchanger/Reactor Heat exchanger/FWR Flow of cooling water to reactor gallons per minute ==
  VPOS(10) : Inport
  VRNG(10) : Inport  Port=2
  " " : Product  Inputs=**/
  Constant2 : Constant  Value=100
  FWR : Outport  VectorParamsAs1DForOutWhenUnconnected=off
  wires:
  Constant2/1 -> " "/3
  " "/1 -> FWR/1
  VPOS(10)/1 -> " "/1
  VRNG(10)/1 -> " "/2

== system COSTEP_Auto/Reactor/Reactor Heat exchanger/Reactor Heat exchanger/Subsystem ==
  VLR : Inport
  Constant : Constant  Value=7.8
  Constant1 : Constant
  Constant2 : Constant  Value=0
  Constant3 : Constant  Value=0.025
  Constant4 : Constant  Value=0.25
  Divide : Product  Inputs=*/
  Divide1 : Product  Inputs=**
  If : If  IfExpression=u1 > 50  ElseIfExpressions=u1 < 10
  If Action Subsystem : Subsystem  TreatAsAtomicUnit=on
  If Action Subsystem1 : Subsystem  TreatAsAtomicUnit=on
  If Action Subsystem2 : Subsystem  TreatAsAtomicUnit=on
  Subtract : Sum  Inputs=+-
  UARLEV : Merge  Inputs=3
  "UARLEV " : Outport  VectorParamsAs1DForOutWhenUnconnected=off
  wires:
  If/2 -> If Action Subsystem1/Action
  If/1 -> If Action Subsystem/Action
  UARLEV/1 -> "UARLEV "/1
  If Action Subsystem1/1(Out1) -> UARLEV/2
  If Action Subsystem/1(Out1) -> UARLEV/1
  If/3 -> If Action Subsystem2/Action
  If Action Subsystem2/1(Out1) -> UARLEV/3
  VLR/1 -> Divide/1
  Constant/1 -> Divide/2
  Divide/1 -> Divide1/2, If/1
  Constant1/1 -> If Action Subsystem/1(In1)
  Constant2/1 -> If Action Subsystem1/1(In1)
  Constant3/1 -> Divide1/1
  Divide1/1 -> Subtract/1
  Constant4/1 -> Subtract/2
  Subtract/1 -> If Action Subsystem2/1(In1)

== system COSTEP_Auto/Reactor/Reactor Heat exchanger/Reactor Heat exchanger/Subsystem2 ==
  UARLEV : Inport
  AGSP : Inport  Port=2
  Add : Sum  Inputs=++-
  Constant : Constant  Value=-0.5
  Constant1 : Constant  Value=2.75
  Constant2 : Constant  Value=2.5
  Constant3 : Constant  Value=855490E-6
  Math Function : Math  Operator=magnitude^2  SignedPower=on
  Product : Product
  Product1 : Product
  UAR : Product  Inputs=3
  "UAR " : Outport
  wires:
  Constant/1 -> Product/1
  Constant3/1 -> UAR/3
  AGSP/1 -> Product1/2, Math Function/1
  Add/1 -> UAR/2
  Product1/1 -> Add/2
  Math Function/1 -> Product/2
  Constant1/1 -> Product1/1
  Constant2/1 -> Add/3
  Product/1 -> Add/1
  UAR/1 -> "UAR "/1
  UARLEV/1 -> UAR/1

== system COSTEP_Auto/Reactor/Reactor Heat exchanger/Reactor Heat exchanger/Subsystem3 ==
  UAR : Inport
  TWR : Inport  Port=2
  TCR : Inport  Port=3
  Bus Selector : BusSelector  OutputSignals=signal2.TESUB8(10)
  Constant4 : Constant
  Constant5 : Constant  Value=0.35
  Product2 : Product
  QUR : Product  Inputs=3
  Subtract : Sum  Inputs=+-
  Subtract1 : Sum  Inputs=+-
  "QUR " : Outport
  wires:
  Product2/1 -> Subtract1/2
  UAR/1 -> QUR/1
  Subtract/1 -> QUR/2
  [TESUB8] -> Bus Selector/1
  Constant4/1 -> Subtract1/1
  Subtract1/1 -> QUR/3
  Constant5/1 -> Product2/1
  TWR/1 -> Subtract/1
  Bus Selector/1 -> Product2/2  "<TESUB8(10)>"
  TCR/1 -> Subtract/2
  QUR/1 -> "QUR "/1

== system COSTEP_Auto/Reactor/Stream 8/Subsystem/If Action Subsystem ==
  In1 : Inport
  Action Port : ActionPort  ActionPortLabel=if(u1 < 0)
  Out1 : Outport  VectorParamsAs1DForOutWhenUnconnected=off
  wires:
  In1/1 -> Out1/1

== system COSTEP_Auto/Reactor/Stream 8/Subsystem/If Action Subsystem1 ==
  In1 : Inport
  Action Port : ActionPort  ActionPortLabel=else
  Out1 : Outport  VectorParamsAs1DForOutWhenUnconnected=off
  wires:
  In1/1 -> Out1/1

== system COSTEP_Auto/Reactor/Volume of Reactor/DLR Molar Density of Liquids in Reactor lb-mol//ft³    /DLR Molar Density of Liquids in Reactor lb-mol//ft³  ==
  X : Inport
  T : Inport  Port=2
  "  " : Constant
  "    " : Product  Inputs=*/
  AD(I) : Constant  Value=AD
  Add2 : Sum
  BD(I) : Constant  Value=BD
  CD(I) : Constant  Value=CD
  Liquid Density of Components lb/ft³ : Sum
  Molecular weight of components lb/lb-mol : Constant  Value=XMW
  Product : Product
  Product1 : Product
  Product2 : Product
  Sum of Elements : Sum  Inputs=+
  V Molar Volume of Components ft³/lb-mol : Product  Inputs=*/
  "R " : Outport  VectorParamsAs1DForOutWhenUnconnected=off
  wires:
  Liquid Density of Components lb/ft³/1 -> V Molar Volume of Components ft³/lb-mol/2
  Product1/1 -> Liquid Density of Components lb/ft³/2
  T/1 -> Product1/2, Product/2
  "  "/1 -> "    "/1
  AD(I)/1 -> Liquid Density of Components lb/ft³/1
  Add2/1 -> Product1/1
  V Molar Volume of Components ft³/lb-mol/1 -> Sum of Elements/1
  CD(I)/1 -> Product/1
  Product2/1 -> V Molar Volume of Components ft³/lb-mol/1
  BD(I)/1 -> Add2/1
  Product/1 -> Add2/2
  "    "/1 -> "R "/1
  X/1 -> Product2/1
  Sum of Elements/1 -> "    "/2
  Molecular weight of components lb/lb-mol/1 -> Product2/2

== system COSTEP_Auto/Separator/Stream 10/Subsystem/If Action Subsystem ==
  In1 : Inport
  Action Port : ActionPort  ActionPortLabel=if(u1 < 0)
  Out1 : Outport  VectorParamsAs1DForOutWhenUnconnected=off
  wires:
  In1/1 -> Out1/1

== system COSTEP_Auto/Separator/Stream 10/Subsystem/If Action Subsystem1 ==
  In1 : Inport
  Action Port : ActionPort  ActionPortLabel=else
  Out1 : Outport  VectorParamsAs1DForOutWhenUnconnected=off
  wires:
  In1/1 -> Out1/1

== system COSTEP_Auto/Separator/Stream 11/PTSL Pressure of Liquid From Separator mmHg/VPR Vapour Pressure mmHg ==
  TCR : Inport
  AVP(I) Antoine Coefficient A ln(mmHg) : Constant  Value=AVP
  Add : Sum
  Add1 : Sum
  BVP(I) Antoine Coefficient B ln(mmHg)·°C : Constant  Value=BVP
  CVP(I) Antoine Coefficient C °C : Constant  Value=CVP
  Divide : Product  Inputs=*/
  Math Function : Math  SignedPower=on
  VPR : Outport  VectorParamsAs1DForOutWhenUnconnected=off
  wires:
  BVP(I) Antoine Coefficient B ln(mmHg)·°C/1 -> Divide/1
  CVP(I) Antoine Coefficient C °C/1 -> Add/1
  AVP(I) Antoine Coefficient A ln(mmHg)/1 -> Add1/1
  Add/1 -> Divide/2
  Divide/1 -> Add1/2
  Add1/1 -> Math Function/1
  Math Function/1 -> VPR/1
  TCR/1 -> Add/2

== system COSTEP_Auto/Separator/Stream 9/Subsystem/If Action Subsystem2 ==
  In1 : Inport
  Action Port : ActionPort  ActionPortLabel=if(u1 < 1E-3)
  Out1 : Outport  VectorParamsAs1DForOutWhenUnconnected=off
  wires:
  In1/1 -> Out1/1

== system COSTEP_Auto/Separator/Stream 9/Subsystem/If Action Subsystem3 ==
  In1 : Inport
  Action Port : ActionPort  ActionPortLabel=else
  Out1 : Outport  PortDimensions=1  VectorParamsAs1DForOutWhenUnconnected=off
  wires:
  In1/1 -> Out1/1

== system COSTEP_Auto/Separator/Stream 9/Subsystem/Pressure drop ==
  Constant : Constant  Value=0.0
  DLP : Sum  Inputs=+-
  DLP Pressure drop between separator and reactor : Merge
  If : If  IfExpression=u1 < 0
  If Action Subsystem : Subsystem  TreatAsAtomicUnit=on
  If Action Subsystem1 : Subsystem  TreatAsAtomicUnit=on
  "DLP " : Outport  VectorParamsAs1DForOutWhenUnconnected=off
  wires:
  DLP Pressure drop between separator and reactor/1 -> "DLP "/1
  [PTV] -> DLP/1
  Constant/1 -> If Action Subsystem/1(In1)
  DLP/1 -> If Action Subsystem1/1(In1), If/1
  If/2 -> If Action Subsystem1/Action
  If/1 -> If Action Subsystem/Action
  [PTS] -> DLP/2
  If Action Subsystem1/1(Out1) -> DLP Pressure drop between separator and reactor/2
  If Action Subsystem/1(Out1) -> DLP Pressure drop between separator and reactor/1

== system COSTEP_Auto/Separator/Volume of Separator/DLS Molar Density of Liquids in Reactor lb-mol//ft³    /DLS Molar Density of Liquids in Separator lb-mol//ft³  ==
  X : Inport
  T : Inport  Port=2
  "  " : Constant
  "    " : Product  Inputs=*/
  AD(I) : Constant  Value=AD
  Add2 : Sum
  BD(I) : Constant  Value=BD
  CD(I) : Constant  Value=CD
  Liquid Density of Components lb/ft³ : Sum
  Product : Product
  Product1 : Product
  Product2 : Product
  Sum of Elements : Sum  Inputs=+
  V Molar Volume of Components ft³/lb-mol : Product  Inputs=*/
  XMW : Constant  Value=XMW
  "R " : Outport  VectorParamsAs1DForOutWhenUnconnected=off
  wires:
  Liquid Density of Components lb/ft³/1 -> V Molar Volume of Components ft³/lb-mol/2
  Product1/1 -> Liquid Density of Components lb/ft³/2
  T/1 -> Product1/2, Product/2
  "  "/1 -> "    "/1
  AD(I)/1 -> Liquid Density of Components lb/ft³/1
  Add2/1 -> Product1/1
  V Molar Volume of Components ft³/lb-mol/1 -> Sum of Elements/1
  CD(I)/1 -> Product/1
  Product2/1 -> V Molar Volume of Components ft³/lb-mol/1
  BD(I)/1 -> Add2/1
  Product/1 -> Add2/2
  "    "/1 -> "R "/1
  X/1 -> Product2/1
  Sum of Elements/1 -> "    "/2
  XMW/1 -> Product2/2

== system COSTEP_Auto/Stream Measurements/Subsystem6/A and C feed stream/Composition measurement mol% ==
  XST : Inport
  XMNSE : Inport  Port=2
  Bus Creator : BusCreator  Inputs=3
  Subsystem : Subsystem
  SMEASX(4) : Outport
  wires:
  Subsystem/3(SMEASXC(4)) -> Bus Creator/3  "SMEASXC(4)"
  XST/1 -> Subsystem/1(XST)
  Subsystem/2(SMEASXB(4)) -> Bus Creator/2  "SMEASXB(4)"
  Subsystem/1(SMEASXA(4)) -> Bus Creator/1  "SMEASXA(4)"
  Bus Creator/1 -> SMEASX(4)/1  "SMEASX(4)"
  XMNSE/1 -> Subsystem/2(XMNSE)

== system COSTEP_Auto/Stream Measurements/Subsystem6/A and C feed stream/Flow measurement in kg//h ==
  XMEAS in kscmh : Inport
  XST : Inport  Port=2
  " " : Constant  Value=35.3145
  "  " : Constant  Value=0.359
  Convert from lb/h to kg/h : Constant  Value=0.454
  Product : Product  Inputs=3
  XMWS Molecular weight of Stream lb/lb-mol : Subsystem
  lb-mol/h : Product  Inputs=**/
  "SMEASF(4) " : Outport  VectorParamsAs1DForOutWhenUnconnected=off
  wires:
  " "/1 -> lb-mol/h/2
  "  "/1 -> lb-mol/h/3
  XMEAS in kscmh/1 -> lb-mol/h/1
  Convert from lb/h to kg/h/1 -> Product/3
  XST/1 -> XMWS Molecular weight of Stream lb/lb-mol/1(XST)
  lb-mol/h/1 -> Product/2
  XMWS Molecular weight of Stream lb/lb-mol/1(XMWS) -> Product/1
  Product/1 -> "SMEASF(4) "/1  "SMEASF(4)"

== system COSTEP_Auto/Stream Measurements/Subsystem6/A and C feed stream/Pressure measurement in kPa ==
  "P in mm Hg " : Inport
  XMNSE : Inport  Port=2
  " kPa" : Constant  Value=101.325
  " mm Hg   " : Constant  Value=760
  Add : Sum
  Pressure conversion kPa : Product  Inputs=*/*
  SMEASP(4) : Outport  VectorParamsAs1DForOutWhenUnconnected=off
  wires:
  "P in mm Hg "/1 -> Pressure conversion kPa/1
  " kPa"/1 -> Pressure conversion kPa/3
  " mm Hg   "/1 -> Pressure conversion kPa/2
  Pressure conversion kPa/1 -> Add/1
  Add/1 -> SMEASP(4)/1  "SMEASP(4)"
  XMNSE/1 -> Add/2

== system COSTEP_Auto/Stream Measurements/Subsystem6/A and C feed stream/Temperature measurement in C ==
  T in celsius : Inport
  XMNSE : Inport  Port=2
  Add : Sum
  SMEAST(4) : Outport
  wires:
  T in celsius/1 -> Add/1
  Add/1 -> SMEAST(4)/1  "SMEAST"
  XMNSE/1 -> Add/2

== system COSTEP_Auto/Stream Measurements/Subsystem6/A feed stream/Composition measurement mol% ==
  XST : Inport
  XMNSE : Inport  Port=2
  Bus Creator : BusCreator  Inputs=2
  Subsystem : Subsystem
  SMEASX(1) : Outport
  wires:
  XST/1 -> Subsystem/1(XST)
  Subsystem/2(SMEASXB(1)) -> Bus Creator/2  "SMEASXB(1)"
  Subsystem/1(SMEASXA(1)) -> Bus Creator/1  "SMEASXA(1)"
  Bus Creator/1 -> SMEASX(1)/1  "SMEASX(1)"
  XMNSE/1 -> Subsystem/2(XMNSE)

== system COSTEP_Auto/Stream Measurements/Subsystem6/A feed stream/Flow measurement in kg//h ==
  XMEAS in kscmh : Inport
  XST : Inport  Port=2
  " " : Constant  Value=35.3145
  "  " : Constant  Value=0.359
  Convert from lb/h to kg/h : Constant  Value=0.454
  XMWS Molecular weight of Stream lb/lb-mol : Subsystem
  kg/h : Product  Inputs=3
  lb-mol/h : Product  Inputs=**/
  "SMEASF(1) " : Outport  VectorParamsAs1DForOutWhenUnconnected=off
  wires:
  " "/1 -> lb-mol/h/2
  "  "/1 -> lb-mol/h/3
  XMEAS in kscmh/1 -> lb-mol/h/1
  Convert from lb/h to kg/h/1 -> kg/h/3
  XST/1 -> XMWS Molecular weight of Stream lb/lb-mol/1(XST)
  lb-mol/h/1 -> kg/h/2
  XMWS Molecular weight of Stream lb/lb-mol/1(XMWS) -> kg/h/1
  kg/h/1 -> "SMEASF(1) "/1

== system COSTEP_Auto/Stream Measurements/Subsystem6/A feed stream/Pressure measurement in kPa ==
  "P in mm Hg " : Inport
  XMNSE : Inport  Port=2
  " kPa" : Constant  Value=101.325
  " mm Hg   " : Constant  Value=760
  Add : Sum
  Pressure conversion kPa : Product  Inputs=*/*
  SMEASP(1) : Outport  VectorParamsAs1DForOutWhenUnconnected=off
  wires:
  "P in mm Hg "/1 -> Pressure conversion kPa/1
  " kPa"/1 -> Pressure conversion kPa/3
  " mm Hg   "/1 -> Pressure conversion kPa/2
  Pressure conversion kPa/1 -> Add/1
  Add/1 -> SMEASP(1)/1  "SMEASP"
  XMNSE/1 -> Add/2

== system COSTEP_Auto/Stream Measurements/Subsystem6/A feed stream/Temperature measurement in C ==
  T in celsius : Inport
  XMNSE : Inport  Port=2
  Add : Sum
  SMEAST(1) : Outport
  wires:
  T in celsius/1 -> Add/1
  Add/1 -> SMEAST(1)/1  "SMEAST"
  XMNSE/1 -> Add/2

== system COSTEP_Auto/Stream Measurements/Subsystem6/CCIn/Flow measurement in kg//h ==
  XMNSE : Inport
  F in gpm : Inport  Port=2
  Add : Sum
  Product : Product
  Product1 : Product
  gpm to lb/h : Constant  Value=500.72
  kg/kmol : Constant  Value=18.02
  kmol : Constant  Value=0.45359237
  kmol/h : Product
  lb/h to lb-mol/h : Product  Inputs=*/
  lb/lb-mol : Constant  Value=18.02
  "SMEASF " : Outport  VectorParamsAs1DForOutWhenUnconnected=off
  wires:
  Add/1 -> "SMEASF "/1  "SMEASF"
  Product/1 -> Add/1
  XMNSE/1 -> Add/2
  Product1/1 -> lb/h to lb-mol/h/1
  lb/lb-mol/1 -> lb/h to lb-mol/h/2
  lb/h to lb-mol/h/1 -> kmol/h/2
  gpm to lb/h/1 -> Product1/2
  F in gpm/1 -> Product1/1
  kmol/1 -> kmol/h/1
  kmol/h/1 -> Product/1
  kg/kmol/1 -> Product/2
